simulink model "Quadrotor_14_step3_noemb"  (Simulink 7.6)
settings: Solver=ode45  StartTime=0.0  StopTime=5000  RelTol=1e-3
undefined symbols (not defined in the file): STARMAC, uav_utilities
libraries: simulink x11, aero_sim_lib x8
(part 2 of 2)

== system Quadrotor_14_step3_noemb/Quadrotor/plant_dynamics/starmac_blade_flapping_effects/starmac_body_moments/CrossProduct(AXB)2 ==
  A : Inport
  B : Inport  Port=2
  Fcn : Fcn  Expr=u[2]*u[6]-u[3]*u[5]
  Fcn1 : Fcn  Expr=u[3]*u[4]-u[1]*u[6]
  Fcn2 : Fcn  Expr=u[1]*u[5]-u[2]*u[4]
  Mux : Mux  Inputs=2
  Mux1 : Mux  Inputs=3
  Out : Outport
  wires:
  Mux1/1 -> Out/1
  Fcn2/1 -> Mux1/3
  Fcn1/1 -> Mux1/2
  Fcn/1 -> Mux1/1
  Mux/1 -> Fcn2/1, Fcn1/1, Fcn/1
  B/1 -> Mux/2
  A/1 -> Mux/1

== system Quadrotor_14_step3_noemb/Quadrotor/plant_dynamics/starmac_blade_flapping_effects/starmac_body_moments/CrossProduct(AXB)3 ==
  A : Inport
  B : Inport  Port=2
  Fcn : Fcn  Expr=u[2]*u[6]-u[3]*u[5]
  Fcn1 : Fcn  Expr=u[3]*u[4]-u[1]*u[6]
  Fcn2 : Fcn  Expr=u[1]*u[5]-u[2]*u[4]
  Mux : Mux  Inputs=2
  Mux1 : Mux  Inputs=3
  Out : Outport
  wires:
  A/1 -> Mux/1
  B/1 -> Mux/2
  Mux/1 -> Fcn/1, Fcn1/1, Fcn2/1
  Fcn/1 -> Mux1/1
  Fcn1/1 -> Mux1/2
  Fcn2/1 -> Mux1/3
  Mux1/1 -> Out/1

== system Quadrotor_14_step3_noemb/Quadrotor/plant_dynamics/starmac_blade_flapping_effects/starmac_body_moments/Motor Thrust to Torques ==
  Thrusts : Inport
  Demux : Demux
  Gain1 : Gain  Gain=K_torque
  torque 1 : Outport
  torque 2 : Outport  Port=2
  torque 3 : Outport  Port=3
  torque 4 : Outport  Port=4
  wires:
  Demux/4 -> torque 4/1
  Demux/3 -> torque 3/1
  Demux/2 -> torque 2/1
  Demux/1 -> torque 1/1
  Gain1/1 -> Demux/1
  Thrusts/1 -> Gain1/1

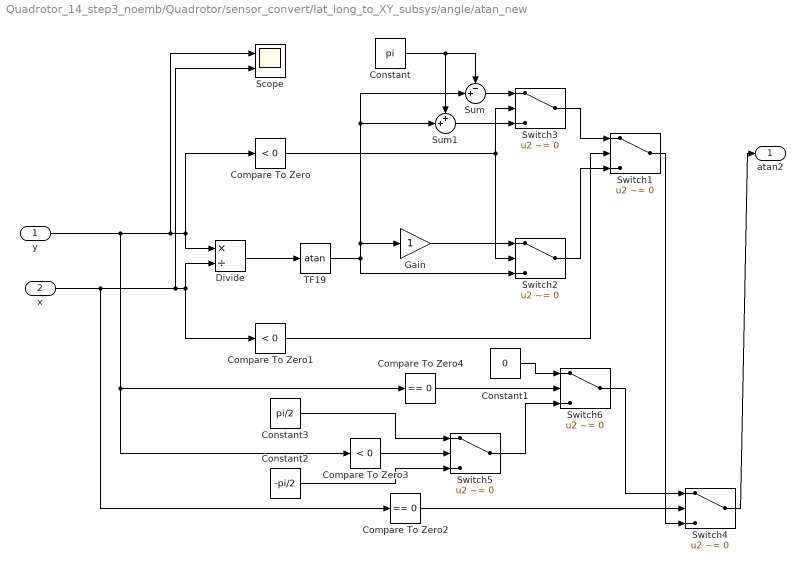
== system Quadrotor_14_step3_noemb/Quadrotor/sensor_convert/lat_long_to_XY_subsys/angle/atan_new ==
  y : Inport
  x : Inport  Port=2
  Compare To Zero : simulink/Logic and Bit Operations/Compare To Zero  SystemSampleTime=-1  relop=<  LogicOutDataTypeMode=uint8
  Compare To Zero1 : simulink/Logic and Bit Operations/Compare To Zero  SystemSampleTime=-1  relop=<  LogicOutDataTypeMode=uint8
  Compare To Zero2 : simulink/Logic and Bit Operations/Compare To Zero  SystemSampleTime=-1  relop===  LogicOutDataTypeMode=uint8
  Compare To Zero3 : simulink/Logic and Bit Operations/Compare To Zero  SystemSampleTime=-1  relop=<  LogicOutDataTypeMode=uint8
  Compare To Zero4 : simulink/Logic and Bit Operations/Compare To Zero  SystemSampleTime=-1  relop===  LogicOutDataTypeMode=uint8
  Constant : Constant  Value=pi
  Constant1 : Constant  Value=0
  Constant2 : Constant  Value=-pi/2
  Constant3 : Constant  Value=pi/2
  Divide : Product  Inputs=*/
  Gain : Gain
  Scope : Scope  NumInputPorts=2
      settings: YMin=-5~-5  YMax=5~5  SaveName=ScopeData2
  Sum : Sum  Inputs=-+|
  Sum1 : Sum  Inputs=++|
  Switch{1..6} (6 alike) : Switch  Criteria=u2 ~= 0
  TF19 : Trigonometry  Operator=atan
  atan2 : Outport
  wires:
  y/1 -> Divide/1, Compare To Zero/1, Scope/1, Compare To Zero4/1, Compare To Zero3/1
  x/1 -> Divide/2, Compare To Zero1/1, Scope/2, Compare To Zero2/1
  Divide/1 -> TF19/1
  Switch2/1 -> Switch1/3
  Switch3/1 -> Switch1/1
  TF19/1 -> Switch2/3, Gain/1, Sum/2, Sum1/2
  Gain/1 -> Switch2/1
  Constant/1 -> Sum1/1, Sum/1
  Sum/1 -> Switch3/1
  Sum1/1 -> Switch3/3
  Compare To Zero/1 -> Switch3/2, Switch2/2
  Compare To Zero1/1 -> Switch1/2
  Compare To Zero2/1 -> Switch4/2
  Compare To Zero3/1 -> Switch5/2
  Compare To Zero4/1 -> Switch6/2
  Switch5/1 -> Switch6/3
  Constant1/1 -> Switch6/1
  Switch6/1 -> Switch4/1
  Switch1/1 -> Switch4/3
  Switch4/1 -> atan2/1
  Constant2/1 -> Switch5/3
  Constant3/1 -> Switch5/1

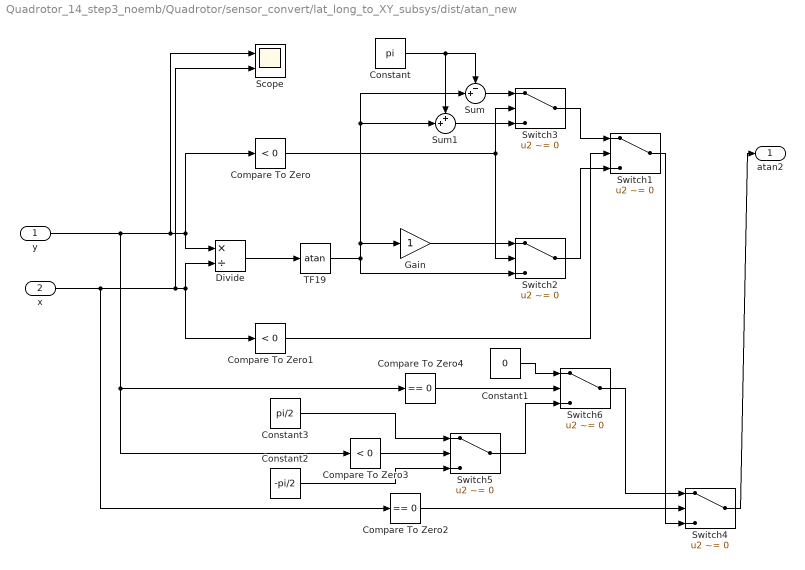
== system Quadrotor_14_step3_noemb/Quadrotor/sensor_convert/lat_long_to_XY_subsys/dist/atan_new ==
  y : Inport
  x : Inport  Port=2
  Compare To Zero : simulink/Logic and Bit Operations/Compare To Zero  SystemSampleTime=-1  relop=<  LogicOutDataTypeMode=uint8
  Compare To Zero1 : simulink/Logic and Bit Operations/Compare To Zero  SystemSampleTime=-1  relop=<  LogicOutDataTypeMode=uint8
  Compare To Zero2 : simulink/Logic and Bit Operations/Compare To Zero  SystemSampleTime=-1  relop===  LogicOutDataTypeMode=uint8
  Compare To Zero3 : simulink/Logic and Bit Operations/Compare To Zero  SystemSampleTime=-1  relop=<  LogicOutDataTypeMode=uint8
  Compare To Zero4 : simulink/Logic and Bit Operations/Compare To Zero  SystemSampleTime=-1  relop===  LogicOutDataTypeMode=uint8
  Constant : Constant  Value=pi
  Constant1 : Constant  Value=0
  Constant2 : Constant  Value=-pi/2
  Constant3 : Constant  Value=pi/2
  Divide : Product  Inputs=*/
  Gain : Gain
  Scope : Scope  NumInputPorts=2
      settings: YMin=-5~-5  YMax=5~5  SaveName=ScopeData2
  Sum : Sum  Inputs=-+|
  Sum1 : Sum  Inputs=++|
  Switch{1..6} (6 alike) : Switch  Criteria=u2 ~= 0
  TF19 : Trigonometry  Operator=atan
  atan2 : Outport
  wires:
  y/1 -> Divide/1, Compare To Zero/1, Scope/1, Compare To Zero4/1, Compare To Zero3/1
  x/1 -> Divide/2, Compare To Zero1/1, Scope/2, Compare To Zero2/1
  Divide/1 -> TF19/1
  Switch2/1 -> Switch1/3
  Switch3/1 -> Switch1/1
  TF19/1 -> Switch2/3, Gain/1, Sum/2, Sum1/2
  Gain/1 -> Switch2/1
  Constant/1 -> Sum1/1, Sum/1
  Sum/1 -> Switch3/1
  Sum1/1 -> Switch3/3
  Compare To Zero/1 -> Switch3/2, Switch2/2
  Compare To Zero1/1 -> Switch1/2
  Compare To Zero2/1 -> Switch4/2
  Compare To Zero3/1 -> Switch5/2
  Compare To Zero4/1 -> Switch6/2
  Switch5/1 -> Switch6/3
  Constant1/1 -> Switch6/1
  Switch6/1 -> Switch4/1
  Switch1/1 -> Switch4/3
  Switch4/1 -> atan2/1
  Constant2/1 -> Switch5/3
  Constant3/1 -> Switch5/1

== matlab function Quadrotor/GPS/XY-to-lat_long/XY-to-lat_long ==
  data: XY input double size=[2]; lat output double; lon output double; lat_0 parameter double; lon_0 parameter double
function [lat,lon] = fcn(XY, lat_0, lon_0)
%Convert inertial X position and Inertial Y position to latitude and
%longitude
    R = 6371e3;          %Earth's Radius meters
    X = XY(1);           %Inertial X position meters
    Y = XY(2);           %Inertial Y position meters
    lat_0 = lat_0*pi/180;
    lon_0 = lon_0*pi/180;
    theta = atan2(Y,X);  %Radians
    d = sqrt(X^2 + Y^2); %Distance from start point (lat_0, lon_0)
    alpha = d/R;
    lat = lat_0 + alpha*cos(theta);
    if abs(theta) == pi/2
        q = cos(lat_0);
    else
        tmp = log(tan((lat/2) + (pi/4))/tan((lat_0/2) + (pi/4)));
        q = alpha*cos(theta)/tmp;
    end
    del_lon = alpha*sin(theta)/q;
    lon = mod((lon_0 + del_lon + pi),2*pi)-pi;
    lat = (180/pi)*lat; %degrees
    lon = (180/pi)*lon; %degrees
    lat = 1e7*lat; %1e-7 degrees
    lon = 1e7*lon; %1e-7 degrees
